simulink model "DumpingSysyemSimulink"  (R2014a)
settings: Solver=ode45  StartTime=0.0  StopTime=100.0  RelTol=1e-3
undefined symbols (not defined in the file or in its folder): B, G, K, M
settings Model: Creator=Kernel  LastModifiedBy=Kernel

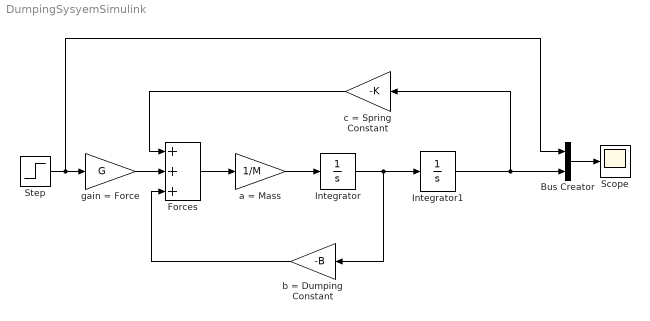
== system DumpingSysyemSimulink ==
  Bus Creator : BusCreator  Inputs=2
  Forces : Sum  Inputs=+++
  Integrator : Integrator
  Integrator1 : Integrator
  Scope : Scope
  Step : Step  SampleTime=0
  a = Mass : Gain  Gain=1/M
  b = Dumping Constant : Gain  Gain=-B
  c = Spring Constant : Gain  Gain=-K
  gain = Force : Gain  Gain=G
  wires:
  Bus Creator/1 -> Scope/1
  Integrator/1 -> b = Dumping Constant/1, Integrator1/1
  b = Dumping Constant/1 -> Forces/3
  c = Spring Constant/1 -> Forces/1
  Forces/1 -> a = Mass/1
  Integrator1/1 -> c = Spring Constant/1, Bus Creator/2
  Step/1 -> Bus Creator/1, gain = Force/1
  a = Mass/1 -> Integrator/1
  gain = Force/1 -> Forces/2
